simulink model "rtp_vector"  (R2020a)
settings: Solver=VariableStepAuto  StartTime=0.0  StopTime=10  RelTol=1e-3
PostLoadFcn:
  | load filters
undefined symbols (not defined in the file): narrow_filter, S, vsva2197, wide_filter, xcvc1902
libraries: ModelComposer x3, simulink x1, dspsrcs4 x1
settings Model: PauseTimes=511  Creator=abehbood  LastModifiedBy=viswanad

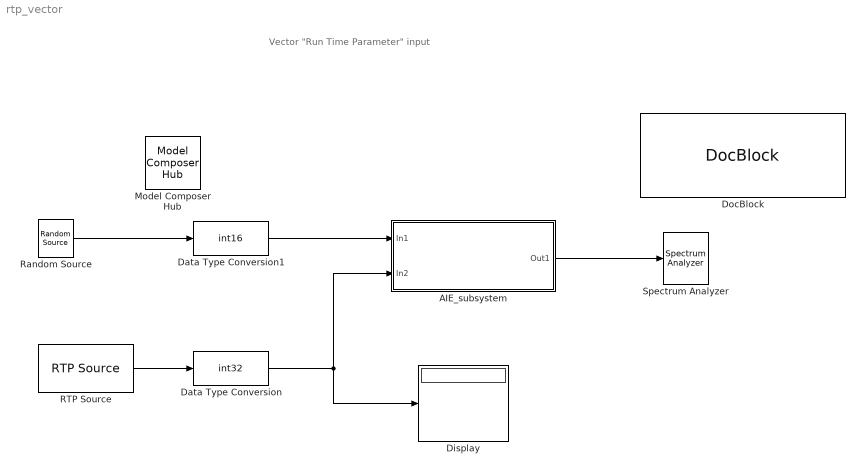
== system rtp_vector ==
  note: Vector "Run Time Parameter" input
  AIE_subsystem : Subsystem
  Data Type Conversion : DataTypeConversion  OutDataTypeStr=int32
  Data Type Conversion1 : DataTypeConversion  OutDataTypeStr=int16
  Display : Display
  DocBlock : simulink/Model-Wide Utilities/DocBlock  DocumentType=Text  mask(DocBlock){}
      content=|
      | ///////////////////////////////////////////////////////////////////////////
      | // Copyright 2020 Xilinx
      | //
      | // Licensed under the Apache License, Version 2.0 (the "License");
      | // you may not use this file except in compliance with the License.
      | // You may obtain a copy of the License at
      | //
      | // http://www.apache.org/licenses/LICENSE-2.0
      | //
      | // Unless required by applicable law or agreed to in writing, software
      | // distributed under the License is distributed on an "AS IS" BASIS,
      | // WITHOUT WARRANTIES OR CONDITIONS OF ANY KIND, either express or implied.
      | // See the License for the specific language governing permissions and
      | // limitations under the License.
      | ///////////////////////////////////////////////////////////////////////////
      mask Display:
      | xmcDrawBlockIcon();
      | disp(['{\fontsize{10pt}(c) Copyright 2020' ' Xilinx, Inc.}\newline \newline '],'texmode','on');
      | disp('{\fontsize{10pt}Licensed under the Apache License 2.0}','texmode','on');
      | disp('\newline \newline \newline{\fontsize{10pt}Double Click for Copyright Notice}','texmode','on');
  Model Composer Hub : ModelComposer/Model Composer Hub  CodeGeneration=off  SubsystemName=AIE_subsystem  TargetDirectory=./code  ExportType=AI Engines  IpVendor=xilinx.com  IpLibrary=hls  IpVersion=1.0  IpHWLanguage=Verilog  AieCompilerOptions={}  CreateTestbench=on  TestbenchStackSize=10  RunAieSim=on  AieSimTimeout=50000  RunAieSimProfiling=off  LaunchVitisAnalyzer=off  PlotOutput=off  RunX86Sim=off  X86SimTimeout=10  PlatformType=Not Specified  ProjDevice=xcvc1902-vsva2197-2MP-e-S  ProjDevicePart=xcvc1902-vsva2197-2MP-e-S  SamplePeriod=-1  ClockFrequency=200  DataPathParallelism=1
  RTP Source : ModelComposer/RTP Source  Value=[repmat(narrow_filter,1, 512), repmat(wide_filter,1, 512)]  SampleTime=-1  OutputForm=Cyclic repetition
  Random Source : dspsrcs4/Random Source  SrcType=Uniform  NormMethod=Ziggurat  CltLength=12  MinVal=-1  MaxVal=1  MeanVal=0  VarVal=1  RepMode=Not repeatable  rawSeed=1  IsInherit=off  SampMode=Discrete  SampTime=1/64  SampFrame=64  DataType=Double  OutComplex=Complex  OutputFrames=off
  Spectrum Analyzer : SpectrumAnalyzer
  wires:
  Data Type Conversion/1 -> AIE_subsystem/2(In2), Display/1
  RTP Source/1 -> Data Type Conversion/1
  Random Source/1 -> Data Type Conversion1/1
  Data Type Conversion1/1 -> AIE_subsystem/1(In1)
  AIE_subsystem/1(Out1) -> Spectrum Analyzer/1

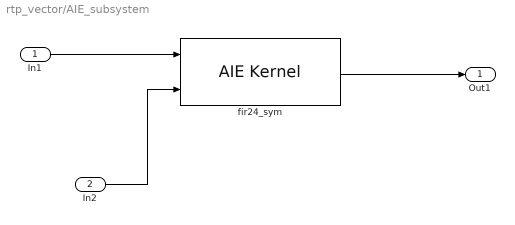
== system rtp_vector/AIE_subsystem ==
  In1 : Inport
  In2 : Inport  Port=2
  fir24_sym : ModelComposer/AIE Kernel  KernelAllAttrs=s[12;12;9;9;19;14;21;23;24;21;12;24;26;26;26;27;28;9;21;23;23;23;24;25;14;19;19;29]@FunctionNameDeclFileNamePortNamesPortTypesPortSerializedTypesPortDirectionsPortWindowSizeEnablesPortWindowMarginEnablesPortSynchronicityEnablesPortSignalSizeEnablesFunctionDeclFunctionTemplateSpecKindFunctionTemplateParamNamesFunctionTemplateParamKindsFunctionTemplateParamTypesFunctionTemplateParamValuesFunctionTemplateParamEnablesClassDeclClassTemplateSpecKindClassTemplateParamNamesClassTemplateParamKindsClassTemplateParamTypesClassTemplateParamValuesClassTemplateParamEnablesClassCtorDeclsClassCtorParamNamesClassCtorParamTypesClassCtorParamSerializedTypes[1 1]@C[28 1]@t9@fir24_symt27@../../src/fir24_sym_param.hC[3 1]@t4@iwint4@owint6@coeffsC[3 1]@t21@input_window_cint16 *t22@output_window_cint16 *t23@int32 const ( &) [ 12 ]C[3 1]@t33@{P{Tinput_window{1{t{Scint16}}}}}t34@{P{Toutput_window{1{t{Scint16}}}}}t18@{R{Q1{C{Bi32}12}}}C[3 1]@t5@inputt6@outputt5@inputC[3 1]@l1@l1@l0@C[3 1]@l1@l0@l0@C[3 1]@l1@l1@l1@C[3 1]@l0@l0@l0@t104@void fir24_sym(input_window_cint16 * iwin, output_window_cint16 * owin, int32 const ( & coeffs ) [ 12 ])t4@nonee[0 1]@e[0 1]@e[0 1]@e[0 1]@e[0 1]@nne[0 1]@e[0 1]@e[0 1]@e[0 1]@e[0 1]@e[0 1]@e[0 1]@e[0 1]@e[0 1]@  PortNames={'iwin'; 'owin'; 'coeffs'}  PortSerializedTypes={'{P{Tinput_window{1{t{Scint16}}}}}'; '{P{Toutput_window{1{t{Scint16}}}}}'; '{R{Q1{C{Bi32}12}}}'}  PortWindowSizes={6.400000000000000000e+01; 6.400000000000000000e+01; 0.000000000000000000e+00}  PortWindowMargins={2.400000000000000000e+01; 0.000000000000000000e+00; 0.000000000000000000e+00}  PortSynchronicities={'sync'; 'auto'; 'sync'}  PortSignalSizes={0.000000000000000000e+00; 0.000000000000000000e+00; 0.000000000000000000e+00}  FunctionTemplateSpecKind=none  FunctionTemplateParamNames={}  FunctionTemplateParamKinds={}  FunctionTemplateParamTypes={}  FunctionTemplateParamValues={}  FunctionIndex=1  FunctionTabVisible=on  FunctionTemplateParamsVisible=off  FunctionDeclTypeOptions=C[1 1]@t104@void fir24_sym(input_window_cint16 * iwin, output_window_cint16 * owin, int32 const ( & coeffs ) [ 12 ])  FunctionDecl=void fir24_sym(input_window_cint16 * iwin, output_window_cint16 * owin, int32 const ( & coeffs ) [ 12 ])  FunctionTemplateParams={}  FunctionTemplateParamsEnables={}  PortAttrs={ 'Input', 'iwin', 'input_window_cint16 *', '64', '24', 'sync', ''; 'Output', 'owin', 'output_window_cint16 *', '64', '', 'auto', ''; 'Input', 'coeffs', 'int32 const ( &) [ 12 ]', '', '', 'sync', '' }  PortAttrsEnables={'off', 'off', 'off', 'on', 'on', 'on', 'off';'off', 'off', 'off', 'on', 'off', 'on', 'off';'off', 'off', 'off', 'off', 'off', 'on', 'off'}  KernelHeaderFile=src/fir24_sym_param.h  KernelFunction=fir24_sym  KernelSourceFile=src/kernels/hb24.cc  KernelSearchPaths={}  PreProcOptions={}  CoreRuntimeRatio=0.5  KernelLocSpec=off  ColRowLocation=[0 0]  blockJsonConstraints=[]  deprecateConstraints=0
  Out1 : Outport
  wires:
  In2/1 -> fir24_sym/2
  In1/1 -> fir24_sym/1
  fir24_sym/1 -> Out1/1
